simulink model "doublePendulum"  (R2013b)
settings: Solver=VariableStepAuto  StartTime=0.0  StopTime=10  RelTol=1e-3
settings Model: Creator=khan  LastModifiedBy=90538
settings DataIOCC: LimitDataPoints=off  SaveFormat=Dataset
settings OptimizationCC: LifeSpan=auto  SimCompilerOptimization=off
settings DebuggingCC: UnderspecifiedInitializationDetection=Simplified  MergeDetectMultiDrivingBlocksExec=error  SolverPrmCheckMsg=none  FcnCallInpInsideContextMsg=error  FrameProcessingCompatibilityMsg=error  SFUnexpectedBacktrackingDiag=error  SFNoUnconditionalDefaultTransitionDiag=error
settings HardwareCC: ProdBitPerPointer=64  ProdLargestAtomicFloat=Float  ProdIntDivRoundTo=Zero  ProdEndianess=LittleEndian  ProdWordSize=64  ProdHWDeviceType=Intel->x86-64 (Windows64)
settings ModelReferenceCC: PropagateSignalLabelsOutOfModel=on
settings RTWCC: RTWCompilerOptimization=off
settings GRTTargetCC: CodeReplacementLibrary=None  GeneratePreprocessorConditionals=Use local settings  CPPClassGenCompliant=on

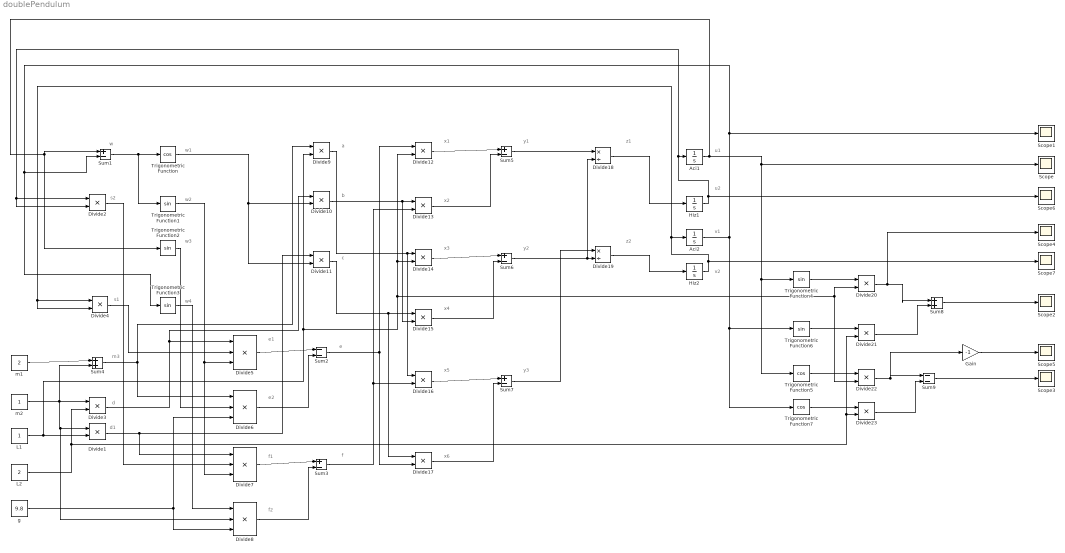
== system doublePendulum ==
  note: w
  note: s2
  note: s1
  note: m3
  note: d
  note: d1
  note: w1
  note: w2
  note: w3
  note: w4
  note: e1
  note: e2
  note: f1
  note: f2
  note: a
  note: b
  note: c
  note: e
  note: f
  note: x1
  note: x2
  note: x3
  note: x4
  note: x5
  note: x6
  note: y1
  note: y2
  note: y3
  note: z1
  note: z2
  note: u2
  note: v2
  note: u1
  note: v1
  Aci1 : Integrator  InitialCondition=pi/3
  Aci2 : Integrator  InitialCondition=3
  Divide{1..4,9..17,20..23} (17 alike) : Product  Inputs=**
  Divide18 : Product  Inputs=*/
  Divide19 : Product  Inputs=*/
  Divide{5..8} (4 alike) : Product  Inputs=***
  Gain : Gain  Gain=-1  SaturateOnIntegerOverflow=off  OutDataTypeStr=Inherit: Inherit via internal rule  ParamDataTypeStr=Inherit: Inherit via internal rule
  Hiz1 : Integrator  InitialCondition=pi/3
  Hiz2 : Integrator
  L1 : Constant
  L2 : Constant  Value=2
  Scope{,1..7} (8 alike) : Scope
      Scope settings: SaveName=Teta1
      Scope1 settings: SaveName=Teta2
      Scope2 settings: SaveName=xTeta2
      Scope3 settings: SaveName=yTeta2
      Scope4 settings: SaveName=xTeta1
      Scope5 settings: SaveName=yTeta1
      Scope6 settings: SaveName=dTeta1dt
      Scope7 settings: SaveName=dTeta2dt
  Sum{1,3,5..7} (5 alike) : Sum  Inputs=|+-
  Sum2 : Sum  Inputs=|--
  Sum4 : Sum  Inputs=|++
  Sum8 : Sum  Inputs=|++
  Sum9 : Sum  Inputs=|--
  Trigonometric Function : Trigonometry  Operator=cos
  Trigonometric Function{1..4,6} (5 alike) : Trigonometry
  Trigonometric Function5 : Trigonometry  Operator=cos
  Trigonometric Function7 : Trigonometry  Operator=cos
  g : Constant  Value=9.8
  m1 : Constant  Value=2
  m2 : Constant
  wires:
  m1/1 -> Sum4/1
  m2/1 -> Divide3/1, Divide8/2, Divide1/1, Sum4/2
  L2/1 -> Divide3/2, Divide21/2, Divide23/2
  L1/1 -> Divide20/2, Divide22/2, Divide14/2, Divide12/2, Divide9/2, Divide1/2
  Sum1/1 -> Trigonometric Function1/1, Trigonometric Function/1
  Divide3/1 -> Divide10/1, Divide5/1
  Divide4/1 -> Divide5/2
  Trigonometric Function1/1 -> Divide7/3, Divide5/3
  g/1 -> Divide8/3, Divide6/3
  Sum4/1 -> Divide9/1, Divide6/1
  Trigonometric Function2/1 -> Divide6/2
  Divide1/1 -> Divide11/1, Divide7/1
  Divide2/1 -> Divide7/2
  Trigonometric Function3/1 -> Divide8/1
  Divide5/1 -> Sum2/1
  Divide6/1 -> Sum2/2
  Divide7/1 -> Sum3/1
  Divide8/1 -> Sum3/2
  Trigonometric Function/1 -> Divide11/2, Divide10/2
  Sum2/1 -> Divide17/2, Divide12/1
  Sum3/1 -> Divide16/2, Divide13/2
  Divide9/1 -> Divide16/1, Divide14/1
  Divide11/1 -> Divide17/1, Divide15/1
  Divide10/1 -> Divide15/2, Divide13/1
  Divide12/1 -> Sum5/1
  Divide13/1 -> Sum5/2
  Divide14/1 -> Sum6/1
  Divide15/1 -> Sum6/2
  Divide16/1 -> Sum7/1
  Divide17/1 -> Sum7/2
  Sum6/1 -> Divide18/2, Divide19/2
  Sum5/1 -> Divide18/1
  Sum7/1 -> Divide19/1
  Divide18/1 -> Hiz1/1
  Divide19/1 -> Hiz2/1
  Hiz1/1 -> Divide2/1, Divide2/2, Aci1/1, Scope6/1
  Hiz2/1 -> Divide4/2, Divide4/1, Aci2/1, Scope7/1
  Aci2/1 -> Trigonometric Function7/1, Trigonometric Function6/1, Scope1/1, Trigonometric Function3/1, Sum1/2
  Aci1/1 -> Trigonometric Function5/1, Trigonometric Function4/1, Scope/1, Sum1/1, Trigonometric Function2/1
  Trigonometric Function4/1 -> Divide20/1
  Trigonometric Function6/1 -> Divide21/1
  Trigonometric Function5/1 -> Divide22/1
  Trigonometric Function7/1 -> Divide23/1
  Divide20/1 -> Scope4/1, Sum8/1
  Divide21/1 -> Sum8/2
  Divide22/1 -> Sum9/1, Gain/1
  Divide23/1 -> Sum9/2
  Sum8/1 -> Scope2/1
  Sum9/1 -> Scope3/1
  Gain/1 -> Scope5/1
